simulink model "SIMULIN_SIMULATION_REFERENCE_FRAME_TRANSFORMATIONS"  (R2020b)
settings: Solver=ode45  StartTime=0.0  StopTime=0.015  RelTol=1e-4  AbsTol=1e-6
settings Model: ModifiedComment=Karim -- Sun Apr 09 01:10:03 2023 -- Version 2.400000e+00  Creator=Karim  LastModifiedBy=Karim
settings Model: ModifiedHistory=|
  | Karim -- Sun Apr 09 01:10:03 2023 -- Version 2.400000e+00
  | 
  | eDrives Embed -- Sun Apr 09 01:09:33 2023 -- Version 2.300000e+00

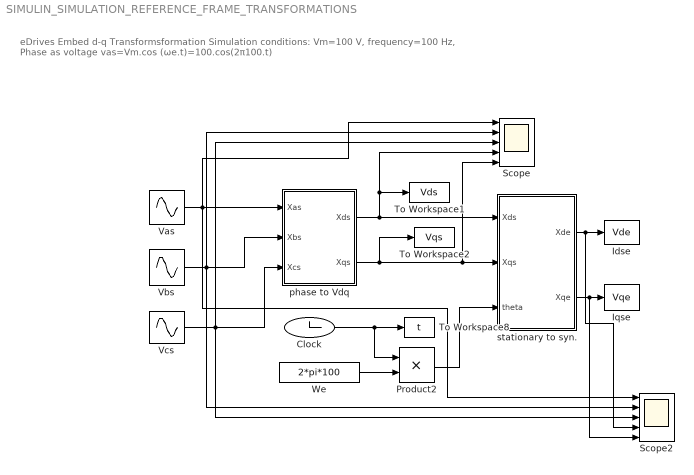
== system SIMULIN_SIMULATION_REFERENCE_FRAME_TRANSFORMATIONS ==
  note: eDrives Embed
      | d-q Transformsformation
      | Simulation conditions: Vm=100 V, frequency=100 Hz,
      | Phase as voltage vas=Vm.cos (ωe.t)=100.cos(2π100.t)
  Clock : Clock
  Idse : ToWorkspace  VariableName=Vde  SampleTime=-1
  Iqse : ToWorkspace  VariableName=Vqe  SampleTime=-1
  Product2 : Product  InputSameDT=on  SaturateOnIntegerOverflow=on  OutDataTypeStr=Inherit: Same as first input
  Scope : Scope  NumInputPorts=5
  Scope2 : Scope  NumInputPorts=5
  To Workspace1 : ToWorkspace  VariableName=Vds  SampleTime=-1
  To Workspace2 : ToWorkspace  VariableName=Vqs  SampleTime=-1
  To Workspace8 : ToWorkspace  VariableName=t  SampleTime=-1
  Vas : Sin  Amplitude=sqrt(2)*100  Frequency=2*pi*100  Phase=pi/2  SampleTime=0
  Vbs : Sin  Amplitude=sqrt(2)*100  Frequency=2*pi*100  Phase=-2/3*pi+pi/2  SampleTime=0
  Vcs : Sin  Amplitude=sqrt(2)*100  Frequency=2*pi*100  Phase=pi/2+2/3*pi  SampleTime=0
  We : Constant  Value=2*pi*100
  phase to Vdq : Subsystem
  stationary to syn. : Subsystem
  wires:
  stationary to syn./2(Xqe) -> Scope2/5, Iqse/1
  stationary to syn./1(Xde) -> Scope2/4, Idse/1
  We/1 -> Product2/2
  phase to Vdq/2(Xqs) -> To Workspace2/1, Scope/5, stationary to syn./2(Xqs)
  Product2/1 -> stationary to syn./3(theta)
  Clock/1 -> To Workspace8/1, Product2/1
  Vas/1 -> Scope2/1, phase to Vdq/1(Xas), Scope/1
  Vbs/1 -> Scope2/2, Scope/2, phase to Vdq/2(Xbs)
  phase to Vdq/1(Xds) -> Scope/4, To Workspace1/1, stationary to syn./1(Xds)
  Vcs/1 -> Scope2/3, Scope/3, phase to Vdq/3(Xcs)

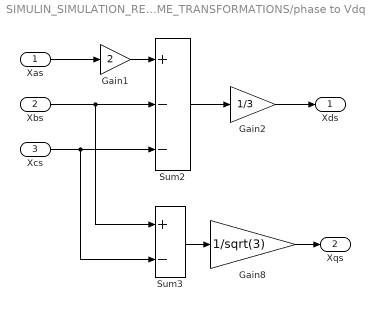
== system SIMULIN_SIMULATION_REFERENCE_FRAME_TRANSFORMATIONS/phase to Vdq ==
  Xas : Inport
  Xbs : Inport  Port=2
  Xcs : Inport  Port=3
  Gain1 : Gain  Gain=2  SaturateOnIntegerOverflow=on  OutDataTypeStr=Inherit: Same as input  ParamDataTypeStr=Inherit: Same as input
  Gain2 : Gain  Gain=1/3  SaturateOnIntegerOverflow=on  OutDataTypeStr=Inherit: Same as input  ParamDataTypeStr=Inherit: Same as input
  Gain8 : Gain  Gain=1/sqrt(3)  SaturateOnIntegerOverflow=on  OutDataTypeStr=Inherit: Same as input  ParamDataTypeStr=Inherit: Same as input
  Sum2 : Sum  Inputs=+--  InputSameDT=on  SaturateOnIntegerOverflow=on  OutDataTypeStr=Inherit: Same as first input
  Sum3 : Sum  Inputs=+-  InputSameDT=on  SaturateOnIntegerOverflow=on  OutDataTypeStr=Inherit: Same as first input
  Xds : Outport  InitialOutput=0
  Xqs : Outport  Port=2  InitialOutput=0
  wires:
  Sum3/1 -> Gain8/1
  Sum2/1 -> Gain2/1
  Xcs/1 -> Sum2/3, Sum3/2
  Xbs/1 -> Sum2/2, Sum3/1
  Xas/1 -> Gain1/1
  Gain1/1 -> Sum2/1
  Gain2/1 -> Xds/1
  Gain8/1 -> Xqs/1

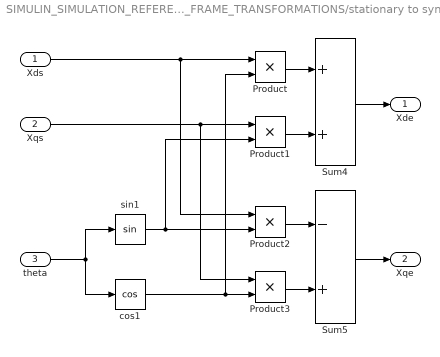
== system SIMULIN_SIMULATION_REFERENCE_FRAME_TRANSFORMATIONS/stationary to syn. ==
  Xds : Inport
  Xqs : Inport  Port=2
  theta : Inport  Port=3
  Product{,1..3} (4 alike) : Product  InputSameDT=on  SaturateOnIntegerOverflow=on  OutDataTypeStr=Inherit: Same as first input
  Sum4 : Sum  InputSameDT=on  SaturateOnIntegerOverflow=on  OutDataTypeStr=Inherit: Same as first input
  Sum5 : Sum  Inputs=-+  InputSameDT=on  SaturateOnIntegerOverflow=on  OutDataTypeStr=Inherit: Same as first input
  cos1 : Trigonometry  Operator=cos
  sin1 : Trigonometry
  Xde : Outport  InitialOutput=0
  Xqe : Outport  Port=2  InitialOutput=0
  wires:
  Product1/1 -> Sum4/2
  Product/1 -> Sum4/1
  Sum4/1 -> Xde/1
  Sum5/1 -> Xqe/1
  Product3/1 -> Sum5/2
  Product2/1 -> Sum5/1
  Xds/1 -> Product2/1, Product/1
  Xqs/1 -> Product3/1, Product1/1
  sin1/1 -> Product2/2, Product1/2
  cos1/1 -> Product3/2, Product/2
  theta/1 -> sin1/1, cos1/1
